simulink library "HEMERO"  (Simulink 3.00)
values from neighbouring files (symbols this model uses):
  K1 = 0.5    [ejh64.m]    (also in ejh65.m)
  K2 = 0.8    [ejh64.m]    (also in ejh65.m)
  x_camino = 0:0.01:10    [ejh64.m]    (also in ejh65.m)
  y_camino = x_camino.^2    [ejh64.m]    (also in ejh65.m)
undefined symbols (not defined in the file or in its folder): magnitude, nonlinear
libraries: simulink_extras x12, HEMERO x9, simulink3 x6, dspstat x4
(part 4 of 9)

== system HEMERO/Robots móviles/Control de robots móviles/Métodos basados en Teoría de Control/Seguimiento de caminos/Seguimiento de caminos (control lineal) ==
  v : Inport  Port=1  PortWidth=-1  SampleTime=-1  DataType=auto
      settings: SignalType=auto
  Configuracion síncrona : Subsystem
  Constant : Constant  Value=x_camino
  Constant1 : Constant  Value=y_camino
  Controlador lineal : Subsystem  Orientation=left
  Convertidor : Subsystem  Orientation=left
      mask Description: Este bloque permite transformar la salida del controlador a una señal que será adecuada al vehículo que se desea controlar
  Cálculo de parámetros : Subsystem
  x_vehículo : Outport  Port=1
  y_vehículo : Outport  Port=2
  phi_vehículo : Outport  Port=3
  wires:
  Constant/1 -> Cálculo de parámetros/1(x_camino)
  Constant1/1 -> Cálculo de parámetros/2(y_camino)
  Cálculo de parámetros/2(fi_gorro) -> Controlador lineal/1(fi_gorro), Convertidor/2(fi_gorro)
  Controlador lineal/1(u_cont) -> Convertidor/4(u_cont)
  Cálculo de parámetros/1(epsilon) -> Controlador lineal/3(epsilon)
  Convertidor/1(w) -> Configuracion síncrona/2(w)
  Configuracion síncrona/1(x_vehículo) -> Cálculo de parámetros/3(x_vehiculo), x_vehículo/1
  Configuracion síncrona/2(y_vehículo) -> Cálculo de parámetros/4(y_vehiculo), y_vehículo/1
  v/1 -> Configuracion síncrona/1(v), Controlador lineal/2(v), Convertidor/3(v)
  Cálculo de parámetros/3(R_c) -> Convertidor/1(R_c)
  Configuracion síncrona/3(phi_vehículo) -> Cálculo de parámetros/5(phi_vehiculo), phi_vehículo/1

== system HEMERO/Robots móviles/Control de robots móviles/Métodos basados en Teoría de Control/Seguimiento de caminos/Seguimiento de caminos (control no lineal) ==
  v : Inport  Port=1  PortWidth=-1  SampleTime=-1  DataType=auto
      settings: SignalType=auto
  " " : Subsystem  Orientation=left  mask{K2=K2}
      mask prompts: K2 "Parámetro K2:"
  Configuracion síncrona : Subsystem
  Constant : Constant  Value=x_camino
  Constant1 : Constant  Value=y_camino
  Controlador no lineal : Subsystem  Orientation=left
  Convertidor : Subsystem  Orientation=left
      mask Description: Este bloque permite transformar la salida del controlador a una señal que será adecuada al vehículo que se desea controlar
  Cálculo de parámetros : Subsystem
  x_vehículo : Outport  Port=1
  y_vehículo : Outport  Port=2
  phi_vehículo : Outport  Port=3
  wires:
  Constant/1 -> Cálculo de parámetros/1(x_camino)
  Constant1/1 -> Cálculo de parámetros/2(y_camino)
  Cálculo de parámetros/2(fi_gorro) -> Controlador no lineal/1(phi_gorro), Convertidor/2(fi_gorro)
  Controlador no lineal/1(u_cont) -> Convertidor/4(u_cont)
  Cálculo de parámetros/1(epsilon) -> Controlador no lineal/3(epsilon)
  Configuracion síncrona/1(x_vehículo) -> Cálculo de parámetros/3(x_vehiculo), x_vehículo/1
  Configuracion síncrona/2(y_vehículo) -> Cálculo de parámetros/4(y_vehiculo), y_vehículo/1
  v/1 -> Configuracion síncrona/1(v), Convertidor/3(v), Controlador no lineal/2(v), " "/1(v)
  Cálculo de parámetros/3(R_c) -> Convertidor/1(R_c)
  " "/1(k (v)) -> Controlador no lineal/4(k (v))
  Configuracion síncrona/3(phi_vehículo) -> Cálculo de parámetros/5(phi_vehiculo), phi_vehículo/1
  Convertidor/1(w) -> Configuracion síncrona/2(w)

== system HEMERO/Robots móviles/Control de robots móviles/Métodos basados en Teoría de Control/Seguimiento de trayectorias/Ejemplos ==
  Ejemplo H.6.6 : Subsystem
  Ejemplo H.6.7 : Subsystem
  Ejemplo H.6.8 : Subsystem

== system HEMERO/Robots móviles/Control de robots móviles/Métodos basados en Teoría de Control/Seguimiento de trayectorias/Seguimiento de trayectorias (Control lineal con escalado de velocidad) ==
  note: v
  note: w
  v_r : Inport  Port=1  PortWidth=-1  SampleTime=-1  DataType=auto
      settings: SignalType=auto
  w_r : Inport  Port=2  PortWidth=-1  SampleTime=-1  DataType=auto
      settings: SignalType=auto
  Cambio de variable : Subsystem
  Configuración síncrona referencia : Subsystem
  Configuración síncrona robot real : Subsystem
  Control lineal con escalado de velocidad : Subsystem
  Product : Product  Inputs=2  SaturateOnIntegerOverflow=on
  Sum : Sum  Inputs=-+  SaturateOnIntegerOverflow=on
  Sum1 : Sum  Inputs=+-  SaturateOnIntegerOverflow=on
  Trigonometric Function : Trigonometry  Operator=cos  OutputSignalType=auto
  v : Outport  Orientation=left  Port=1
  w : Outport  Orientation=left  Port=2
  x_ref : Outport  Port=3
  x : Outport  Port=4
  y_ref : Outport  Port=5
  y : Outport  Port=6
  phi_ref : Outport  Port=7
  phi : Outport  Port=8
  wires:
  v_r/1 -> Configuración síncrona referencia/1(v_r), Product/2, Control lineal con escalado de velocidad/4(v_r)
  Trigonometric Function/1 -> Product/1
  Product/1 -> Sum/2
  w_r/1 -> Configuración síncrona referencia/2(w_r), Sum1/1, Control lineal con escalado de velocidad/5(w_r)
  Sum1/1 -> Configuración síncrona robot real/2(w), w/1
  Sum/1 -> Configuración síncrona robot real/1(v), v/1
  Control lineal con escalado de velocidad/2(u2) -> Sum1/2
  Control lineal con escalado de velocidad/1(u1) -> Sum/1
  Cambio de variable/1(e1) -> Control lineal con escalado de velocidad/1(e1)
  Cambio de variable/2(e2) -> Control lineal con escalado de velocidad/2(e2)
  Cambio de variable/3(e3) -> Trigonometric Function/1, Control lineal con escalado de velocidad/3(e3)
  Configuración síncrona robot real/3(phi) -> Cambio de variable/6(phi), phi/1
  Configuración síncrona referencia/3(phi_r) -> Cambio de variable/5(phi_r), phi_ref/1
  Configuración síncrona robot real/2(y) -> Cambio de variable/4(y), y/1
  Configuración síncrona referencia/2(y_r) -> Cambio de variable/3(y_r), y_ref/1
  Configuración síncrona robot real/1(x) -> Cambio de variable/2(x), x/1
  Configuración síncrona referencia/1(x_r) -> Cambio de variable/1(x_r), x_ref/1

== system HEMERO/Robots móviles/Control de robots móviles/Métodos basados en Teoría de Control/Seguimiento de trayectorias/Seguimiento de trayectorias (Control lineal) ==
  note: v
  note: w
  v_r : Inport  Port=1  PortWidth=-1  SampleTime=-1  DataType=auto
      settings: SignalType=auto
  w_r : Inport  Port=2  PortWidth=-1  SampleTime=-1  DataType=auto
      settings: SignalType=auto
  Cambio de variable : Subsystem
  Configuración síncrona referencia : Subsystem
  Configuración síncrona robot real : Subsystem
  Control lineal : Subsystem
  Product : Product  Inputs=2  SaturateOnIntegerOverflow=on
  Sum : Sum  Inputs=-+  SaturateOnIntegerOverflow=on
  Sum1 : Sum  Inputs=+-  SaturateOnIntegerOverflow=on
  Trigonometric Function : Trigonometry  Operator=cos  OutputSignalType=auto
  v : Outport  Orientation=left  Port=1
  w : Outport  Orientation=left  Port=2
  x_ref : Outport  Port=3
  x : Outport  Port=4
  y_ref : Outport  Port=5
  y : Outport  Port=6
  phi_ref : Outport  Port=7
  phi : Outport  Port=8
  wires:
  v_r/1 -> Configuración síncrona referencia/1(v_r), Product/2, Control lineal/4(v_r)
  Trigonometric Function/1 -> Product/1
  Product/1 -> Sum/2
  w_r/1 -> Configuración síncrona referencia/2(w_r), Sum1/1
  Sum1/1 -> Configuración síncrona robot real/2(w), w/1
  Sum/1 -> Configuración síncrona robot real/1(v), v/1
  Control lineal/2(u2) -> Sum1/2
  Control lineal/1(u1) -> Sum/1
  Cambio de variable/1(e1) -> Control lineal/1(e1)
  Cambio de variable/2(e2) -> Control lineal/2(e2)
  Cambio de variable/3(e3) -> Trigonometric Function/1, Control lineal/3(e3)
  Configuración síncrona referencia/1(x_r) -> Cambio de variable/1(x_r), x_ref/1
  Configuración síncrona robot real/1(x) -> Cambio de variable/2(x), x/1
  Configuración síncrona referencia/2(y_r) -> Cambio de variable/3(y_r), y_ref/1
  Configuración síncrona robot real/2(y) -> Cambio de variable/4(y), y/1
  Configuración síncrona referencia/3(phi_r) -> Cambio de variable/5(phi_r), phi_ref/1
  Configuración síncrona robot real/3(phi) -> Cambio de variable/6(phi), phi/1

== system HEMERO/Robots móviles/Control de robots móviles/Métodos basados en Teoría de Control/Seguimiento de trayectorias/Seguimiento de trayectorias (Control no lineal) ==
  note: v
  note: w
  v_r : Inport  Port=1  PortWidth=-1  SampleTime=-1  DataType=auto
      settings: SignalType=auto
  w_r : Inport  Port=2  PortWidth=-1  SampleTime=-1  DataType=auto
      settings: SignalType=auto
  " " : Trigonometry  Operator=cos  OutputSignalType=auto
  Cambio de variable : Subsystem
  Configuración síncrona referencia : Subsystem
  Configuración síncrona robot real : Subsystem
  Control no lineal : Subsystem
  Cálculo de K1 y K3 : Subsystem
  Product : Product  Inputs=2  SaturateOnIntegerOverflow=on
  Sum : Sum  Inputs=-+  SaturateOnIntegerOverflow=on
  Sum1 : Sum  Inputs=+-  SaturateOnIntegerOverflow=on
  v : Outport  Orientation=left  Port=1
  w : Outport  Orientation=left  Port=2
  x_ref : Outport  Port=3
  x : Outport  Port=4
  y_ref : Outport  Port=5
  y : Outport  Port=6
  phi_ref : Outport  Port=7
  phi : Outport  Port=8
  wires:
  v_r/1 -> Configuración síncrona referencia/1(v_r), Product/2, Control no lineal/4(v_r), Cálculo de K1 y K3/2(v_r)
  " "/1 -> Product/1
  Product/1 -> Sum/2
  w_r/1 -> Configuración síncrona referencia/2(w_r), Sum1/1, Cálculo de K1 y K3/1(w_r)
  Sum1/1 -> Configuración síncrona robot real/2(w), w/1
  Sum/1 -> Configuración síncrona robot real/1(v), v/1
  Control no lineal/2(u2) -> Sum1/2
  Control no lineal/1(u1) -> Sum/1
  Cambio de variable/1(e1) -> Control no lineal/1(e1)
  Cambio de variable/2(e2) -> Control no lineal/2(e2)
  Cambio de variable/3(e3) -> " "/1, Control no lineal/3(e3)
  Cálculo de K1 y K3/1(K1) -> Control no lineal/5(K1), Control no lineal/6(K3)
  Configuración síncrona robot real/3(phi) -> Cambio de variable/6(phi), phi/1
  Configuración síncrona referencia/1(x_r) -> Cambio de variable/1(x_r), x_ref/1
  Configuración síncrona robot real/1(x) -> Cambio de variable/2(x), x/1
  Configuración síncrona referencia/2(y_r) -> Cambio de variable/3(y_r), y_ref/1
  Configuración síncrona robot real/2(y) -> Cambio de variable/4(y), y/1
  Configuración síncrona referencia/3(phi_r) -> Cambio de variable/5(phi_r), phi_ref/1

== system HEMERO/Robots manipuladores base fija/Control basado en el modelo/Control Adaptativo/Ejemplos/Ejemplo H.5.5/Control PD ==
  qd : Inport  Port=1  PortWidth=-1  SampleTime=-1  DataType=auto
      settings: SignalType=auto
  q : Inport  Port=2  PortWidth=-1  SampleTime=-1  DataType=auto
      settings: SignalType=auto
  qd' : Inport  Port=3  PortWidth=-1  SampleTime=-1  DataType=auto
      settings: SignalType=auto
  q' : Inport  Port=4  PortWidth=-1  SampleTime=-1  DataType=auto
      settings: SignalType=auto
  A : StateSpace  A=[]  B=[]  C=[]  D=K  X0=0  mask(Matrix Gain){@1=A}
      mask prompts: @1 "Gain matrix:"
      mask help: Matrix Gain.
      mask init:
      | K=@1;
      mask Help: Multiplies input vector by entered matrix to produce output vector (y=Au).
      mask Display: disp('K')
  Kv : StateSpace  A=[]  B=[]  C=[]  D=K  X0=0  mask(Matrix Gain){@1=Kv}
      mask prompts: @1 "Gain matrix:"
      mask help: Matrix Gain.
      mask init:
      | K=@1;
      mask Help: Multiplies input vector by entered matrix to produce output vector (y=Au).
      mask Display: disp('K')
  Kv1 : StateSpace  A=[]  B=[]  C=[]  D=K  X0=0  mask(Matrix Gain){@1=Kv}
      mask prompts: @1 "Gain matrix:"
      mask help: Matrix Gain.
      mask init:
      | K=@1;
      mask Help: Multiplies input vector by entered matrix to produce output vector (y=Au).
      mask Display: disp('K')
  Sum : Sum  Inputs=+-  SaturateOnIntegerOverflow=on
  Sum1 : Sum  Inputs=+-  SaturateOnIntegerOverflow=on
  Sum2 : Sum  Inputs=++  SaturateOnIntegerOverflow=on
  tau_r : Outport  Port=1  InitialOutput=0
  wires:
  Sum2/1 -> tau_r/1
  Kv1/1 -> Sum2/1
  Kv/1 -> Sum2/2
  Sum1/1 -> Kv/1
  q'/1 -> Sum1/2
  qd'/1 -> Sum1/1
  q/1 -> Sum/2
  qd/1 -> Sum/1
  Sum/1 -> A/1
  A/1 -> Kv1/1

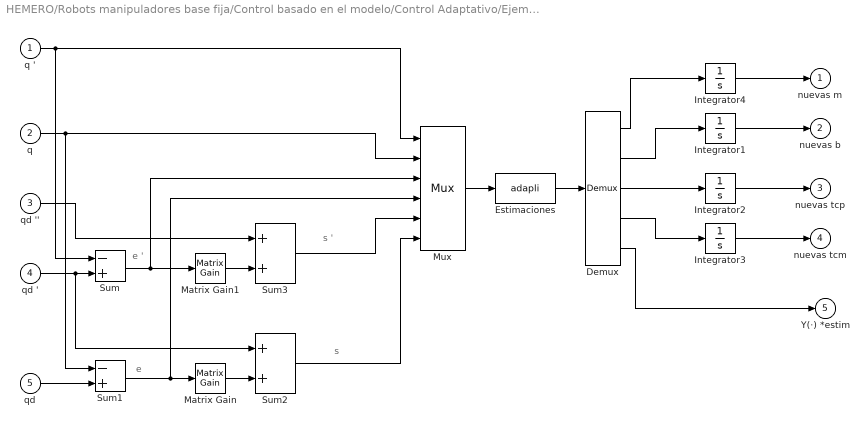
== system HEMERO/Robots manipuladores base fija/Control basado en el modelo/Control Adaptativo/Ejemplos/Ejemplo H.5.5/Control de inercia adaptativo ==
  note: e
  note: e '
  note: s
  note: s '
  q ' : Inport  Port=1  PortWidth=-1  SampleTime=-1  DataType=auto
      settings: SignalType=auto
  q : Inport  Port=2  PortWidth=-1  SampleTime=-1  DataType=auto
      settings: SignalType=auto
  qd '' : Inport  Port=3  PortWidth=-1  SampleTime=-1  DataType=auto
      settings: SignalType=auto
  qd ' : Inport  Port=4  PortWidth=-1  SampleTime=-1  DataType=auto
      settings: SignalType=auto
  qd : Inport  Port=5  PortWidth=-1  SampleTime=-1  DataType=auto
      settings: SignalType=auto
  Demux : Demux  Outputs=5
  Estimaciones : S-Function  FunctionName=adapli  Parameters=dyn, gamma, a, grav  PortCounts=[]  SFunctionModules=''
  Integrator1 : Integrator  ExternalReset=none  InitialConditionSource=internal  InitialCondition=b_inicial(:)  LimitOutput=off  UpperSaturationLimit=inf  LowerSaturationLimit=-inf  ShowSaturationPort=off  ShowStatePort=off  AbsoluteTolerance=auto
  Integrator2 : Integrator  ExternalReset=none  InitialConditionSource=internal  InitialCondition=tcp_inicial(:)  LimitOutput=off  UpperSaturationLimit=inf  LowerSaturationLimit=-inf  ShowSaturationPort=off  ShowStatePort=off  AbsoluteTolerance=auto
  Integrator3 : Integrator  ExternalReset=none  InitialConditionSource=internal  InitialCondition=tcm_inicial(:)  LimitOutput=off  UpperSaturationLimit=inf  LowerSaturationLimit=-inf  ShowSaturationPort=off  ShowStatePort=off  AbsoluteTolerance=auto
  Integrator4 : Integrator  ExternalReset=none  InitialConditionSource=internal  InitialCondition=m_inicial(:)  LimitOutput=off  UpperSaturationLimit=inf  LowerSaturationLimit=-inf  ShowSaturationPort=off  ShowStatePort=off  AbsoluteTolerance=auto
  Matrix Gain : simulink3/Math/Matrix Gain  K=a
  Matrix Gain1 : simulink3/Math/Matrix Gain  K=a
  Mux : Mux  Inputs=6
      settings: DisplayOption=none
  Sum : Sum  Inputs=-+  SaturateOnIntegerOverflow=on
  Sum1 : Sum  Inputs=-+  SaturateOnIntegerOverflow=on
  Sum2 : Sum  Inputs=++  SaturateOnIntegerOverflow=on
  Sum3 : Sum  Inputs=++  SaturateOnIntegerOverflow=on
  nuevas m : Outport  Port=1  InitialOutput=0
  nuevas b : Outport  Port=2  InitialOutput=0
  nuevas tcp : Outport  Port=3  InitialOutput=0
  nuevas tcm : Outport  Port=4  InitialOutput=0
  Y(·) *estim : Outport  Port=5  InitialOutput=0
  wires:
  q '/1 -> Mux/1, Sum/1
  q/1 -> Mux/2, Sum1/1
  Mux/1 -> Estimaciones/1
  Estimaciones/1 -> Demux/1
  Demux/2 -> Integrator1/1
  Integrator1/1 -> nuevas b/1
  Demux/3 -> Integrator2/1
  Integrator2/1 -> nuevas tcp/1
  Demux/4 -> Integrator3/1
  Integrator3/1 -> nuevas tcm/1
  qd/1 -> Sum1/2
  Matrix Gain/1 -> Sum2/2
  qd '/1 -> Sum/2, Sum2/1
  Matrix Gain1/1 -> Sum3/2
  qd ''/1 -> Sum3/1
  Sum2/1 -> Mux/6
  Sum3/1 -> Mux/5
  Sum/1 -> Matrix Gain1/1, Mux/3
  Sum1/1 -> Matrix Gain/1, Mux/4
  Demux/5 -> Y(·) *estim/1
  Demux/1 -> Integrator4/1
  Integrator4/1 -> nuevas m/1

== system HEMERO/Robots manipuladores base fija/Control basado en el modelo/Control Adaptativo/Ejemplos/Ejemplo H.5.5/Inversa de la matriz de masas real ==
  q : Inport  Port=1  PortWidth=-1  SampleTime=-1  DataType=auto
      settings: SignalType=auto
  In : Inport  Port=2  PortWidth=-1  SampleTime=-1  DataType=auto
      settings: SignalType=auto
  Masas : S-Function  FunctionName=sminv  Parameters=dyn  PortCounts=[]  SFunctionModules=''
  Mux : Mux  Inputs=2
      settings: DisplayOption=none
  M(q)^(-1) · In : Outport  Port=1  InitialOutput=0
  wires:
  Mux/1 -> Masas/1
  q/1 -> Mux/1
  In/1 -> Mux/2
  Masas/1 -> M(q)^(-1) · In/1

== system HEMERO/Robots manipuladores base fija/Control basado en el modelo/Control Adaptativo/Ejemplos/Ejemplo H.5.5/Término gravitatorio estimado ==
  q : Inport  Port=1  PortWidth=-1  SampleTime=-1  DataType=auto
      settings: SignalType=auto
  nuevas m : Inport  Port=2  PortWidth=-1  SampleTime=-1  DataType=auto
      settings: SignalType=auto
  Gravedad : S-Function  FunctionName=esgravity  Parameters=dyn,grav  PortCounts=[]  SFunctionModules=''
  Mux : Mux  Inputs=2
      settings: DisplayOption=none
  G (q) : Outport  Port=1  InitialOutput=0
  wires:
  Mux/1 -> Gravedad/1
  nuevas m/1 -> Mux/2
  q/1 -> Mux/1
  Gravedad/1 -> G (q)/1

== system HEMERO/Robots manipuladores base fija/Control basado en el modelo/Control Adaptativo/Ejemplos/Ejemplo H.5.5/Término gravitatorio real ==
  q : Inport  Port=1  PortWidth=-1  SampleTime=-1  DataType=auto
      settings: SignalType=auto
  Gravedad : S-Function  FunctionName=sgravity  Parameters=dyn,grav  PortCounts=[]  SFunctionModules=''
  G (q) : Outport  Port=1  InitialOutput=0
  wires:
  q/1 -> Gravedad/1
  Gravedad/1 -> G (q)/1

== system HEMERO/Robots manipuladores base fija/Control basado en el modelo/Control Adaptativo/Ejemplos/Ejemplo H.5.5/Término Vm de Coriolis estimado ==
  q : Inport  Port=1  PortWidth=-1  SampleTime=-1  DataType=auto
      settings: SignalType=auto
  q ' : Inport  Port=2  PortWidth=-1  SampleTime=-1  DataType=auto
      settings: SignalType=auto
  In : Inport  Port=3  PortWidth=-1  SampleTime=-1  DataType=auto
      settings: SignalType=auto
  nuevas m : Inport  Port=4  PortWidth=-1  SampleTime=-1  DataType=auto
      settings: SignalType=auto
  "  " : S-Function  FunctionName=esvmcorioli  Parameters=dyn  PortCounts=[]  SFunctionModules=''
  Mux : Mux  Inputs=4
      settings: DisplayOption=none
  Vm (q,q')·In : Outport  Port=1  InitialOutput=0
  wires:
  nuevas m/1 -> Mux/4
  "  "/1 -> Vm (q,q')·In/1
  Mux/1 -> "  "/1
  In/1 -> Mux/3
  q/1 -> Mux/1
  q '/1 -> Mux/2

== system HEMERO/Robots manipuladores base fija/Control basado en el modelo/Control Adaptativo/Ejemplos/Ejemplo H.5.5/Término de la matriz de masas estimado ==
  q : Inport  Port=1  PortWidth=-1  SampleTime=-1  DataType=auto
      settings: SignalType=auto
  In : Inport  Port=2  PortWidth=-1  SampleTime=-1  DataType=auto
      settings: SignalType=auto
  nuevas m : Inport  Port=3  PortWidth=-1  SampleTime=-1  DataType=auto
      settings: SignalType=auto
  Masas : S-Function  FunctionName=esinertia  Parameters=dyn  PortCounts=[]  SFunctionModules=''
  Mux : Mux  Inputs=3
      settings: DisplayOption=none
  M (q)·In : Outport  Port=1  InitialOutput=0
  wires:
  nuevas m/1 -> Mux/3
  Masas/1 -> M (q)·In/1
  Mux/1 -> Masas/1
  q/1 -> Mux/1
  In/1 -> Mux/2

== system HEMERO/Robots manipuladores base fija/Control basado en el modelo/Control Adaptativo/Ejemplos/Ejemplo H.5.5/Términos centrífugos y de Coriolis reales ==
  q : Inport  Port=1  PortWidth=-1  SampleTime=-1  DataType=auto
      settings: SignalType=auto
  q' : Inport  Port=2  PortWidth=-1  SampleTime=-1  DataType=auto
      settings: SignalType=auto
  Centrífugos y Coriolis : S-Function  FunctionName=scoriolis  Parameters=dyn  PortCounts=[]  SFunctionModules=''
  Mux : Mux  Inputs=2
      settings: DisplayOption=none
  V (q,q') : Outport  Port=1  InitialOutput=0
  wires:
  Mux/1 -> Centrífugos y Coriolis/1
  q/1 -> Mux/1
  q'/1 -> Mux/2
  Centrífugos y Coriolis/1 -> V (q,q')/1

== system HEMERO/Robots manipuladores base fija/Control basado en el modelo/Control con aprendizaje/Ejemplos/Ejemplo H.5.1/Control PD ==
  qd : Inport  Port=1  PortWidth=-1  SampleTime=-1  DataType=auto
      settings: SignalType=auto
  q : Inport  Port=2  PortWidth=-1  SampleTime=-1  DataType=auto
      settings: SignalType=auto
  qd' : Inport  Port=3  PortWidth=-1  SampleTime=-1  DataType=auto
      settings: SignalType=auto
  q' : Inport  Port=4  PortWidth=-1  SampleTime=-1  DataType=auto
      settings: SignalType=auto
  qd'' : Inport  Port=5  PortWidth=-1  SampleTime=-1  DataType=auto
      settings: SignalType=auto
  Kp : StateSpace  A=[]  B=[]  C=[]  D=K  X0=0  mask(Matrix Gain){@1=Kp}
      mask prompts: @1 "Gain matrix:"
      mask help: Matrix Gain.
      mask init:
      | K=@1;
      mask Help: Multiplies input vector by entered matrix to produce output vector (y=Au).
      mask Display: disp('K')
  Kv : StateSpace  A=[]  B=[]  C=[]  D=K  X0=0  mask(Matrix Gain){@1=Kv}
      mask prompts: @1 "Gain matrix:"
      mask help: Matrix Gain.
      mask init:
      | K=@1;
      mask Help: Multiplies input vector by entered matrix to produce output vector (y=Au).
      mask Display: disp('K')
  Sum : Sum  Inputs=+-  SaturateOnIntegerOverflow=on
  Sum1 : Sum  Inputs=+-  SaturateOnIntegerOverflow=on
  Sum2 : Sum  Inputs=+++  SaturateOnIntegerOverflow=on
  tau_r : Outport  Port=1  InitialOutput=0
  wires:
  Sum2/1 -> tau_r/1
  qd''/1 -> Sum2/3
  Kp/1 -> Sum2/1
  Kv/1 -> Sum2/2
  Sum1/1 -> Kv/1
  Sum/1 -> Kp/1
  q'/1 -> Sum1/2
  qd'/1 -> Sum1/1
  q/1 -> Sum/2
  qd/1 -> Sum/1

== system HEMERO/Robots manipuladores base fija/Control basado en el modelo/Control con aprendizaje/Ejemplos/Ejemplo H.5.1/Modelo del robot ==
  note: q
  note: q''
  note: q'
  tau : Inport  Port=1  PortWidth=-1  SampleTime=-1  DataType=auto
      settings: SignalType=auto
  Integrator : Integrator  ExternalReset=none  InitialConditionSource=internal  InitialCondition=inivel(:)  LimitOutput=off  UpperSaturationLimit=inf  LowerSaturationLimit=-inf  ShowSaturationPort=off  ShowStatePort=off  AbsoluteTolerance=auto
  Integrator1 : Integrator  ExternalReset=none  InitialConditionSource=internal  InitialCondition=inipos(:)  LimitOutput=off  UpperSaturationLimit=inf  LowerSaturationLimit=-inf  ShowSaturationPort=off  ShowStatePort=off  AbsoluteTolerance=auto
  Inversa de la matriz de masas : HEMERO/Robots manipuladores base fija/Modelo Dinámico/Trayectorias articulares/Inversa de la matriz de masas  dyn=dyn
  Modelo de fricciones : HEMERO/Robots manipuladores base fija/Modelo Dinámico/Trayectorias articulares/Modelo de fricciones  G=dyn (:,17)  b=dyn (:,18)  tcp=dyn (:,19)  tcm=dyn (:,20)
  Sum : Sum  Inputs=+---  SaturateOnIntegerOverflow=on
  Términos gravitatorios : HEMERO/Robots manipuladores base fija/Modelo Dinámico/Trayectorias articulares/Términos gravitatorios  dyn=dyn  grav=grav
  Términos centrífugos y de Coriolis : HEMERO/Robots manipuladores base fija/Modelo Dinámico/Trayectorias articulares/Términos centrífugos y de Coriolis  dyn=dyn
  q : Outport  Port=1  InitialOutput=0
  q' : Outport  Port=2  InitialOutput=0
  q'' : Outport  Port=3  InitialOutput=0
  wires:
  Integrator1/1 -> q/1, Inversa de la matriz de masas/1, Términos centrífugos y de Coriolis/1, Términos gravitatorios/1
  Integrator/1 -> Integrator1/1, q'/1, Términos centrífugos y de Coriolis/2, Modelo de fricciones/1
  Sum/1 -> Inversa de la matriz de masas/2
  tau/1 -> Sum/1
  Inversa de la matriz de masas/1 -> Integrator/1, q''/1
  Términos gravitatorios/1 -> Sum/4
  Términos centrífugos y de Coriolis/1 -> Sum/3
  Modelo de fricciones/1 -> Sum/2

== system HEMERO/Robots manipuladores base fija/Control basado en el modelo/Control con aprendizaje/Ejemplos/Ejemplo H.5.1/Par realimentado aprendido ==
  note: e ''
  note: e '
  note: e
  qd '' : Inport  Port=1  PortWidth=-1  SampleTime=-1  DataType=auto
      settings: SignalType=auto
  q '' : Inport  Port=2  PortWidth=-1  SampleTime=-1  DataType=auto
      settings: SignalType=auto
  qd ' : Inport  Port=3  PortWidth=-1  SampleTime=-1  DataType=auto
      settings: SignalType=auto
  q ' : Inport  Port=4  PortWidth=-1  SampleTime=-1  DataType=auto
      settings: SignalType=auto
  qd : Inport  Port=5  PortWidth=-1  SampleTime=-1  DataType=auto
      settings: SignalType=auto
  q : Inport  Port=6  PortWidth=-1  SampleTime=-1  DataType=auto
      settings: SignalType=auto
  Demux : Demux  Outputs=4
  Mux : Mux  Inputs=3
      settings: DisplayOption=none
  S-Function : S-Function  FunctionName=learn  Parameters=Kp, Kv, mu, tfinal  PortCounts=[]  SFunctionModules=''
  Sum : Sum  Inputs=+-  SaturateOnIntegerOverflow=on
  Sum1 : Sum  Inputs=+-  SaturateOnIntegerOverflow=on
  Sum2 : Sum  Inputs=+-  SaturateOnIntegerOverflow=on
  To Workspace1 : ToWorkspace  VariableName=error  SampleTime=-1  SaveFormat=Matrix
  To Workspace2 : ToWorkspace  VariableName=error_d  SampleTime=-1  SaveFormat=Matrix
  To Workspace3 : ToWorkspace  VariableName=error_dd  SampleTime=-1  SaveFormat=Matrix
  To Workspace4 : ToWorkspace  VariableName=edd  SampleTime=-1  SaveFormat=Matrix
  To Workspace5 : ToWorkspace  VariableName=dknueva  SampleTime=-1  SaveFormat=Matrix
  To Workspace6 : ToWorkspace  VariableName=ed  SampleTime=-1  SaveFormat=Matrix
  To Workspace7 : ToWorkspace  VariableName=e  SampleTime=-1  SaveFormat=Matrix
  Término de la matriz de masas estimado : Subsystem  mask(Término asociado a la matriz de masas){dyn=dyn}
      mask prompts: dyn "Matriz de parámetros cinemáticos y dinámicos:"
      mask help: Este bloque calcula el par correspondiente al término en el que aparece la matriz de masas.
  gamma (k) : Outport  Port=1
  wires:
  Mux/1 -> S-Function/1
  S-Function/1 -> Demux/1
  qd ''/1 -> Sum/1
  q ''/1 -> Sum/2
  qd '/1 -> Sum1/1
  q '/1 -> Sum1/2
  qd/1 -> Sum2/1
  Demux/1 -> Término de la matriz de masas estimado/2(In), To Workspace5/1
  Sum2/1 -> Mux/3, To Workspace7/1
  Sum1/1 -> Mux/2, To Workspace6/1
  Sum/1 -> Mux/1, To Workspace4/1
  Demux/2 -> To Workspace1/1
  Demux/3 -> To Workspace2/1
  Demux/4 -> To Workspace3/1
  q/1 -> Sum2/2, Término de la matriz de masas estimado/1(q)
  Término de la matriz de masas estimado/1(M (q)·In) -> gamma (k)/1

== system HEMERO/Robots manipuladores base fija/Control basado en el modelo/Control con aprendizaje/Ejemplos/Ejemplo H.5.1/Término de la matriz de masas ==
  q : Inport  Port=1  PortWidth=-1  SampleTime=-1  DataType=auto
      settings: SignalType=auto
  In : Inport  Port=2  PortWidth=-1  SampleTime=-1  DataType=auto
      settings: SignalType=auto
  Masas : S-Function  FunctionName=sinertia  Parameters=dyn  PortCounts=[]  SFunctionModules=''
  Mux : Mux  Inputs=2
      settings: DisplayOption=none
  M (q)·In : Outport  Port=1  InitialOutput=0
  wires:
  Masas/1 -> M (q)·In/1
  In/1 -> Mux/2
  q/1 -> Mux/1
  Mux/1 -> Masas/1

== system HEMERO/Robots manipuladores base fija/Control basado en el modelo/Control con aprendizaje/Ejemplos/Ejemplo H.5.1/Términos gravitatorios ==
  q : Inport  Port=1  PortWidth=-1  SampleTime=-1  DataType=auto
      settings: SignalType=auto
  Gravedad : S-Function  FunctionName=sgravity  Parameters=dyn,grav  PortCounts=[]  SFunctionModules=''
  G (q) : Outport  Port=1  InitialOutput=0
  wires:
  Gravedad/1 -> G (q)/1
  q/1 -> Gravedad/1

== system HEMERO/Robots manipuladores base fija/Control basado en el modelo/Control con aprendizaje/Ejemplos/Ejemplo H.5.1/Términos centrífugos y de Coriolis ==
  q : Inport  Port=1  PortWidth=-1  SampleTime=-1  DataType=auto
      settings: SignalType=auto
  q' : Inport  Port=2  PortWidth=-1  SampleTime=-1  DataType=auto
      settings: SignalType=auto
  Centrífugos y Coriolis : S-Function  FunctionName=scoriolis  Parameters=dyn  PortCounts=[]  SFunctionModules=''
  Mux : Mux  Inputs=2
      settings: DisplayOption=none
  V (q,q') : Outport  Port=1  InitialOutput=0
  wires:
  Centrífugos y Coriolis/1 -> V (q,q')/1
  q'/1 -> Mux/2
  q/1 -> Mux/1
  Mux/1 -> Centrífugos y Coriolis/1

== system HEMERO/Robots manipuladores base fija/Control basado en el modelo/Par Computado/Ejemplos/Ejemplo H.5.2/Control PD ==
  qd : Inport  Port=1  PortWidth=-1  SampleTime=-1  DataType=auto
      settings: SignalType=auto
  q : Inport  Port=2  PortWidth=-1  SampleTime=-1  DataType=auto
      settings: SignalType=auto
  qd' : Inport  Port=3  PortWidth=-1  SampleTime=-1  DataType=auto
      settings: SignalType=auto
  q' : Inport  Port=4  PortWidth=-1  SampleTime=-1  DataType=auto
      settings: SignalType=auto
  qd'' : Inport  Port=5  PortWidth=-1  SampleTime=-1  DataType=auto
      settings: SignalType=auto
  Kp : StateSpace  A=[]  B=[]  C=[]  D=K  X0=0  mask(Matrix Gain){@1=Kp}
      mask prompts: @1 "Gain matrix:"
      mask help: Matrix Gain.
      mask init:
      | K=@1;
      mask Help: Multiplies input vector by entered matrix to produce output vector (y=Au).
      mask Display: disp('K')
  Kv : StateSpace  A=[]  B=[]  C=[]  D=K  X0=0  mask(Matrix Gain){@1=Kv}
      mask prompts: @1 "Gain matrix:"
      mask help: Matrix Gain.
      mask init:
      | K=@1;
      mask Help: Multiplies input vector by entered matrix to produce output vector (y=Au).
      mask Display: disp('K')
  Sum : Sum  Inputs=+-  SaturateOnIntegerOverflow=on
  Sum1 : Sum  Inputs=+-  SaturateOnIntegerOverflow=on
  Sum2 : Sum  Inputs=+++  SaturateOnIntegerOverflow=on
  tau_r : Outport  Port=1  InitialOutput=0
  wires:
  qd/1 -> Sum/1
  q/1 -> Sum/2
  qd'/1 -> Sum1/1
  q'/1 -> Sum1/2
  Sum/1 -> Kp/1
  Sum1/1 -> Kv/1
  Kv/1 -> Sum2/2
  Kp/1 -> Sum2/1
  qd''/1 -> Sum2/3
  Sum2/1 -> tau_r/1

== system HEMERO/Robots manipuladores base fija/Control basado en el modelo/Par Computado/Ejemplos/Ejemplo H.5.2/Estimada1 ==
  q : Inport  Port=1  PortWidth=-1  SampleTime=-1  DataType=auto
      settings: SignalType=auto
  Gravedad : S-Function  FunctionName=sgravity  Parameters=dyn,grav  PortCounts=[]  SFunctionModules=''
  G (q) : Outport  Port=1  InitialOutput=0
  wires:
  q/1 -> Gravedad/1
  Gravedad/1 -> G (q)/1

== system HEMERO/Robots manipuladores base fija/Control basado en el modelo/Par Computado/Ejemplos/Ejemplo H.5.2/Estimada2 ==
  q : Inport  Port=1  PortWidth=-1  SampleTime=-1  DataType=auto
      settings: SignalType=auto
  In : Inport  Port=2  PortWidth=-1  SampleTime=-1  DataType=auto
      settings: SignalType=auto
  Masas : S-Function  FunctionName=sinertia  Parameters=dyn  PortCounts=[]  SFunctionModules=''
  Mux : Mux  Inputs=2
      settings: DisplayOption=none
  M (q)·In : Outport  Port=1  InitialOutput=0
  wires:
  Mux/1 -> Masas/1
  q/1 -> Mux/1
  In/1 -> Mux/2
  Masas/1 -> M (q)·In/1

== system HEMERO/Robots manipuladores base fija/Control basado en el modelo/Par Computado/Ejemplos/Ejemplo H.5.2/Estimada3 ==
  q : Inport  Port=1  PortWidth=-1  SampleTime=-1  DataType=auto
      settings: SignalType=auto
  q' : Inport  Port=2  PortWidth=-1  SampleTime=-1  DataType=auto
      settings: SignalType=auto
  Centrífugos y Coriolis : S-Function  FunctionName=scoriolis  Parameters=dyn  PortCounts=[]  SFunctionModules=''
  Mux : Mux  Inputs=2
      settings: DisplayOption=none
  V (q,q') : Outport  Port=1  InitialOutput=0
  wires:
  Mux/1 -> Centrífugos y Coriolis/1
  q/1 -> Mux/1
  q'/1 -> Mux/2
  Centrífugos y Coriolis/1 -> V (q,q')/1

== system HEMERO/Robots manipuladores base fija/Control basado en el modelo/Par Computado/Ejemplos/Ejemplo H.5.2/Real1 ==
  q : Inport  Port=1  PortWidth=-1  SampleTime=-1  DataType=auto
      settings: SignalType=auto
  q' : Inport  Port=2  PortWidth=-1  SampleTime=-1  DataType=auto
      settings: SignalType=auto
  Centrífugos y Coriolis : S-Function  FunctionName=scoriolis  Parameters=dyn  PortCounts=[]  SFunctionModules=''
  Mux : Mux  Inputs=2
      settings: DisplayOption=none
  V (q,q') : Outport  Port=1  InitialOutput=0
  wires:
  Mux/1 -> Centrífugos y Coriolis/1
  q/1 -> Mux/1
  q'/1 -> Mux/2
  Centrífugos y Coriolis/1 -> V (q,q')/1

== system HEMERO/Robots manipuladores base fija/Control basado en el modelo/Par Computado/Ejemplos/Ejemplo H.5.2/Real2 ==
  q : Inport  Port=1  PortWidth=-1  SampleTime=-1  DataType=auto
      settings: SignalType=auto
  Gravedad : S-Function  FunctionName=sgravity  Parameters=dyn,grav  PortCounts=[]  SFunctionModules=''
  G (q) : Outport  Port=1  InitialOutput=0
  wires:
  q/1 -> Gravedad/1
  Gravedad/1 -> G (q)/1

== system HEMERO/Robots manipuladores base fija/Control basado en el modelo/Par Computado/Ejemplos/Ejemplo H.5.2/Real3 ==
  q : Inport  Port=1  PortWidth=-1  SampleTime=-1  DataType=auto
      settings: SignalType=auto
  In : Inport  Port=2  PortWidth=-1  SampleTime=-1  DataType=auto
      settings: SignalType=auto
  Masas : S-Function  FunctionName=sminv  Parameters=dyn  PortCounts=[]  SFunctionModules=''
  Mux : Mux  Inputs=2
      settings: DisplayOption=none
  M(q)^(-1) · In : Outport  Port=1  InitialOutput=0
  wires:
  Mux/1 -> Masas/1
  q/1 -> Mux/1
  In/1 -> Mux/2
  Masas/1 -> M(q)^(-1) · In/1

== system HEMERO/Robots manipuladores base fija/Control basado en el modelo/Par Computado/Ejemplos/Ejemplo H.5.3/Control PD ==
  qd : Inport  Port=1  PortWidth=-1  SampleTime=-1  DataType=auto
      settings: SignalType=auto
  q : Inport  Port=2  PortWidth=-1  SampleTime=-1  DataType=auto
      settings: SignalType=auto
  qd' : Inport  Port=3  PortWidth=-1  SampleTime=-1  DataType=auto
      settings: SignalType=auto
  q' : Inport  Port=4  PortWidth=-1  SampleTime=-1  DataType=auto
      settings: SignalType=auto
  qd'' : Inport  Port=5  PortWidth=-1  SampleTime=-1  DataType=auto
      settings: SignalType=auto
  Kp : HEMERO/Robots manipuladores base fija/Control basado en el modelo/Par Computado/Ejemplos/Ejemplo H.5.2/Control PD/Kp  MaskParam1=Kp
  Kv : HEMERO/Robots manipuladores base fija/Control basado en el modelo/Par Computado/Ejemplos/Ejemplo H.5.2/Control PD/Kv  MaskParam1=Kv
  Sum : Sum  Inputs=+-  SaturateOnIntegerOverflow=on
  Sum1 : Sum  Inputs=+-  SaturateOnIntegerOverflow=on
  Sum2 : Sum  Inputs=+++  SaturateOnIntegerOverflow=on
  tau_r : Outport  Port=1  InitialOutput=0
  wires:
  qd/1 -> Sum/1
  q/1 -> Sum/2
  qd'/1 -> Sum1/1
  q'/1 -> Sum1/2
  Sum/1 -> Kp/1
  Sum1/1 -> Kv/1
  Kv/1 -> Sum2/2
  Kp/1 -> Sum2/1
  qd''/1 -> Sum2/3
  Sum2/1 -> tau_r/1

== system HEMERO/Robots manipuladores base fija/Control basado en el modelo/Par Computado/Ejemplos/Ejemplo H.5.3/Estimada1 ==
  q : Inport  Port=1  PortWidth=-1  SampleTime=-1  DataType=auto
      settings: SignalType=auto
  Gravedad : S-Function  FunctionName=sgravity  Parameters=dyn,grav  PortCounts=[]  SFunctionModules=''
  G (q) : Outport  Port=1  InitialOutput=0
  wires:
  q/1 -> Gravedad/1
  Gravedad/1 -> G (q)/1

== system HEMERO/Robots manipuladores base fija/Control basado en el modelo/Par Computado/Ejemplos/Ejemplo H.5.3/Estimada2 ==
  q : Inport  Port=1  PortWidth=-1  SampleTime=-1  DataType=auto
      settings: SignalType=auto
  In : Inport  Port=2  PortWidth=-1  SampleTime=-1  DataType=auto
      settings: SignalType=auto
  Masas : S-Function  FunctionName=sinertia  Parameters=dyn  PortCounts=[]  SFunctionModules=''
  Mux : Mux  Inputs=2
      settings: DisplayOption=none
  M (q)·In : Outport  Port=1  InitialOutput=0
  wires:
  Mux/1 -> Masas/1
  q/1 -> Mux/1
  In/1 -> Mux/2
  Masas/1 -> M (q)·In/1

== system HEMERO/Robots manipuladores base fija/Control basado en el modelo/Par Computado/Ejemplos/Ejemplo H.5.3/Estimada3 ==
  q : Inport  Port=1  PortWidth=-1  SampleTime=-1  DataType=auto
      settings: SignalType=auto
  q' : Inport  Port=2  PortWidth=-1  SampleTime=-1  DataType=auto
      settings: SignalType=auto
  Centrífugos y Coriolis : S-Function  FunctionName=scoriolis  Parameters=dyn  PortCounts=[]  SFunctionModules=''
  Mux : Mux  Inputs=2
      settings: DisplayOption=none
  V (q,q') : Outport  Port=1  InitialOutput=0
  wires:
  Mux/1 -> Centrífugos y Coriolis/1
  q/1 -> Mux/1
  q'/1 -> Mux/2
  Centrífugos y Coriolis/1 -> V (q,q')/1

== system HEMERO/Robots manipuladores base fija/Control basado en el modelo/Par Computado/Ejemplos/Ejemplo H.5.3/Real1 ==
  q : Inport  Port=1  PortWidth=-1  SampleTime=-1  DataType=auto
      settings: SignalType=auto
  q' : Inport  Port=2  PortWidth=-1  SampleTime=-1  DataType=auto
      settings: SignalType=auto
  Centrífugos y Coriolis : S-Function  FunctionName=scoriolis  Parameters=dyn  PortCounts=[]  SFunctionModules=''
  Mux : Mux  Inputs=2
      settings: DisplayOption=none
  V (q,q') : Outport  Port=1  InitialOutput=0
  wires:
  Mux/1 -> Centrífugos y Coriolis/1
  q/1 -> Mux/1
  q'/1 -> Mux/2
  Centrífugos y Coriolis/1 -> V (q,q')/1

== system HEMERO/Robots manipuladores base fija/Control basado en el modelo/Par Computado/Ejemplos/Ejemplo H.5.3/Real2 ==
  q : Inport  Port=1  PortWidth=-1  SampleTime=-1  DataType=auto
      settings: SignalType=auto
  Gravedad : S-Function  FunctionName=sgravity  Parameters=dyn,grav  PortCounts=[]  SFunctionModules=''
  G (q) : Outport  Port=1  InitialOutput=0
  wires:
  q/1 -> Gravedad/1
  Gravedad/1 -> G (q)/1

== system HEMERO/Robots manipuladores base fija/Control basado en el modelo/Par Computado/Ejemplos/Ejemplo H.5.3/Real3 ==
  q : Inport  Port=1  PortWidth=-1  SampleTime=-1  DataType=auto
      settings: SignalType=auto
  In : Inport  Port=2  PortWidth=-1  SampleTime=-1  DataType=auto
      settings: SignalType=auto
  Masas : S-Function  FunctionName=sminv  Parameters=dyn  PortCounts=[]  SFunctionModules=''
  Mux : Mux  Inputs=2
      settings: DisplayOption=none
  M(q)^(-1) · In : Outport  Port=1  InitialOutput=0
  wires:
  Mux/1 -> Masas/1
  q/1 -> Mux/1
  In/1 -> Mux/2
  Masas/1 -> M(q)^(-1) · In/1

== system HEMERO/Robots manipuladores base fija/Control basado en el modelo/Par Computado/Ejemplos/Ejemplo H.5.4/Control PID ==
  note: e
  note: e'
  qd : Inport  Port=1  PortWidth=-1  SampleTime=-1  DataType=auto
      settings: SignalType=auto
  q : Inport  Port=2  PortWidth=-1  SampleTime=-1  DataType=auto
      settings: SignalType=auto
  qd' : Inport  Port=3  PortWidth=-1  SampleTime=-1  DataType=auto
      settings: SignalType=auto
  q' : Inport  Port=4  PortWidth=-1  SampleTime=-1  DataType=auto
      settings: SignalType=auto
  qd'' : Inport  Port=5  PortWidth=-1  SampleTime=-1  DataType=auto
      settings: SignalType=auto
  Integrator : Integrator  ExternalReset=none  InitialConditionSource=internal  InitialCondition=0  LimitOutput=off  UpperSaturationLimit=inf  LowerSaturationLimit=-inf  ShowSaturationPort=off  ShowStatePort=off  AbsoluteTolerance=auto
  Ki : HEMERO/Robots manipuladores base fija/Control basado en el modelo/Par Computado/Control PID/Ki  MaskParam1=Ki
  Kp : HEMERO/Robots manipuladores base fija/Control basado en el modelo/Par Computado/Control PID/Kp  MaskParam1=Kp
  Kv : HEMERO/Robots manipuladores base fija/Control basado en el modelo/Par Computado/Control PID/Kv  MaskParam1=Kv
  Sum : Sum  Inputs=+-  SaturateOnIntegerOverflow=on
  Sum1 : Sum  Inputs=+-  SaturateOnIntegerOverflow=on
  Sum2 : Sum  Inputs=++++  SaturateOnIntegerOverflow=on
  tau_r : Outport  Port=1  InitialOutput=0
  wires:
  Sum2/1 -> tau_r/1
  Sum1/1 -> Kv/1
  q'/1 -> Sum1/2
  qd'/1 -> Sum1/1
  q/1 -> Sum/2
  qd/1 -> Sum/1
  qd''/1 -> Sum2/4
  Kv/1 -> Sum2/3
  Kp/1 -> Sum2/2
  Sum/1 -> Kp/1, Ki/1
  Ki/1 -> Integrator/1
  Integrator/1 -> Sum2/1

== system HEMERO/Robots manipuladores base fija/Control basado en el modelo/Par Computado/Ejemplos/Ejemplo H.5.4/Estimada1 ==
  q : Inport  Port=1  PortWidth=-1  SampleTime=-1  DataType=auto
      settings: SignalType=auto
  Gravedad : S-Function  FunctionName=sgravity  Parameters=dyn,grav  PortCounts=[]  SFunctionModules=''
  G (q) : Outport  Port=1  InitialOutput=0
  wires:
  q/1 -> Gravedad/1
  Gravedad/1 -> G (q)/1

== system HEMERO/Robots manipuladores base fija/Control basado en el modelo/Par Computado/Ejemplos/Ejemplo H.5.4/Estimada2 ==
  q : Inport  Port=1  PortWidth=-1  SampleTime=-1  DataType=auto
      settings: SignalType=auto
  In : Inport  Port=2  PortWidth=-1  SampleTime=-1  DataType=auto
      settings: SignalType=auto
  Masas : S-Function  FunctionName=sinertia  Parameters=dyn  PortCounts=[]  SFunctionModules=''
  Mux : Mux  Inputs=2
      settings: DisplayOption=none
  M (q)·In : Outport  Port=1  InitialOutput=0
  wires:
  Mux/1 -> Masas/1
  q/1 -> Mux/1
  In/1 -> Mux/2
  Masas/1 -> M (q)·In/1

== system HEMERO/Robots manipuladores base fija/Control basado en el modelo/Par Computado/Ejemplos/Ejemplo H.5.4/Estimada3 ==
  q : Inport  Port=1  PortWidth=-1  SampleTime=-1  DataType=auto
      settings: SignalType=auto
  q' : Inport  Port=2  PortWidth=-1  SampleTime=-1  DataType=auto
      settings: SignalType=auto
  Centrífugos y Coriolis : S-Function  FunctionName=scoriolis  Parameters=dyn  PortCounts=[]  SFunctionModules=''
  Mux : Mux  Inputs=2
      settings: DisplayOption=none
  V (q,q') : Outport  Port=1  InitialOutput=0
  wires:
  Mux/1 -> Centrífugos y Coriolis/1
  q/1 -> Mux/1
  q'/1 -> Mux/2
  Centrífugos y Coriolis/1 -> V (q,q')/1

== system HEMERO/Robots manipuladores base fija/Control basado en el modelo/Par Computado/Ejemplos/Ejemplo H.5.4/Real1 ==
  q : Inport  Port=1  PortWidth=-1  SampleTime=-1  DataType=auto
      settings: SignalType=auto
  q' : Inport  Port=2  PortWidth=-1  SampleTime=-1  DataType=auto
      settings: SignalType=auto
  Centrífugos y Coriolis : S-Function  FunctionName=scoriolis  Parameters=dyn  PortCounts=[]  SFunctionModules=''
  Mux : Mux  Inputs=2
      settings: DisplayOption=none
  V (q,q') : Outport  Port=1  InitialOutput=0
  wires:
  Mux/1 -> Centrífugos y Coriolis/1
  q/1 -> Mux/1
  q'/1 -> Mux/2
  Centrífugos y Coriolis/1 -> V (q,q')/1

== system HEMERO/Robots manipuladores base fija/Control basado en el modelo/Par Computado/Ejemplos/Ejemplo H.5.4/Real2 ==
  q : Inport  Port=1  PortWidth=-1  SampleTime=-1  DataType=auto
      settings: SignalType=auto
  Gravedad : S-Function  FunctionName=sgravity  Parameters=dyn,grav  PortCounts=[]  SFunctionModules=''
  G (q) : Outport  Port=1  InitialOutput=0
  wires:
  q/1 -> Gravedad/1
  Gravedad/1 -> G (q)/1

== system HEMERO/Robots manipuladores base fija/Control basado en el modelo/Par Computado/Ejemplos/Ejemplo H.5.4/Real3 ==
  q : Inport  Port=1  PortWidth=-1  SampleTime=-1  DataType=auto
      settings: SignalType=auto
  In : Inport  Port=2  PortWidth=-1  SampleTime=-1  DataType=auto
      settings: SignalType=auto
  Masas : S-Function  FunctionName=sminv  Parameters=dyn  PortCounts=[]  SFunctionModules=''
  Mux : Mux  Inputs=2
      settings: DisplayOption=none
  M(q)^(-1) · In : Outport  Port=1  InitialOutput=0
  wires:
  Mux/1 -> Masas/1
  q/1 -> Mux/1
  In/1 -> Mux/2
  Masas/1 -> M(q)^(-1) · In/1

== system HEMERO/Robots manipuladores base fija/Modelo Dinámico/Ejemplos/Ejemplo H.4.2/Trayectorias articulares/Inversa de la matriz de masas ==
  q : Inport  Port=1  PortWidth=-1  SampleTime=-1  DataType=auto
      settings: SignalType=auto
  In : Inport  Port=2  PortWidth=-1  SampleTime=-1  DataType=auto
      settings: SignalType=auto
  Masas : S-Function  FunctionName=sminv  Parameters=dyn  PortCounts=[]  SFunctionModules=''
  Mux : Mux  Inputs=2
      settings: DisplayOption=none
  M(q)^(-1) · In : Outport  Port=1  InitialOutput=0
  wires:
  Masas/1 -> M(q)^(-1) · In/1
  In/1 -> Mux/2
  q/1 -> Mux/1
  Mux/1 -> Masas/1

== system HEMERO/Robots manipuladores base fija/Modelo Dinámico/Ejemplos/Ejemplo H.4.2/Trayectorias articulares/Modelo de fricciones ==
  q' : Inport  Port=1  PortWidth=-1  SampleTime=-1  DataType=auto
      settings: SignalType=auto
  Fricciones : S-Function  FunctionName=sfriction  Parameters=G,b,tcp,tcm  PortCounts=[]  SFunctionModules=''
  tau_f : Outport  Port=1  InitialOutput=0
  wires:
  Fricciones/1 -> tau_f/1
  q'/1 -> Fricciones/1

== system HEMERO/Robots manipuladores base fija/Modelo Dinámico/Ejemplos/Ejemplo H.4.2/Trayectorias articulares/Términos gravitatorios ==
  q : Inport  Port=1  PortWidth=-1  SampleTime=-1  DataType=auto
      settings: SignalType=auto
  Gravedad : S-Function  FunctionName=sgravity  Parameters=dyn,grav  PortCounts=[]  SFunctionModules=''
  G (q) : Outport  Port=1  InitialOutput=0
  wires:
  Gravedad/1 -> G (q)/1
  q/1 -> Gravedad/1

== system HEMERO/Robots manipuladores base fija/Modelo Dinámico/Ejemplos/Ejemplo H.4.2/Trayectorias articulares/Términos centrífugos y de Coriolis ==
  q : Inport  Port=1  PortWidth=-1  SampleTime=-1  DataType=auto
      settings: SignalType=auto
  q' : Inport  Port=2  PortWidth=-1  SampleTime=-1  DataType=auto
      settings: SignalType=auto
  Centrífugos y Coriolis : S-Function  FunctionName=scoriolis  Parameters=dyn  PortCounts=[]  SFunctionModules=''
  Mux : Mux  Inputs=2
      settings: DisplayOption=none
  V (q,q') : Outport  Port=1  InitialOutput=0
  wires:
  Centrífugos y Coriolis/1 -> V (q,q')/1
  q'/1 -> Mux/2
  q/1 -> Mux/1
  Mux/1 -> Centrífugos y Coriolis/1

== system HEMERO/Robots móviles/Control de robots móviles/Métodos basados en Teoría de Control/Seguimiento de caminos/Ejemplos/Ejemplo H.6.4 ==
  Constant1 : Constant  Value=1
  Seguimiento de caminos (control lineal) : Subsystem  mask(Seguimiento de caminos empleando una ley de control lineal){x_inicial=0, y_inicial=0, phi_inicial=0, K1=K1, K2=K2, x_camino=x_camino, y_camino=y_camino}
      mask prompts: x_inicial "Coordenada x inicial del móvil:"; y_inicial "Coordenada y inicial del móvil:"; phi_inicial "Valor inicial de la orientación del móvil:"; K1 "Parámetro K1:"; K2 "Parámetro K2:"; x_camino "Vector con las coordenadas x del camino:"; y_camino "Vector con las coordenadas y del camino:"
      mask help:
      | Este bloque permite simular una estrategia de control lineal para el seguimiento de caminos.
      | A la entrada se dispone de la velocidad del vehículo en cada instante y mediante los parámetros es posible introducir las coordenadas (x,y) del camino. A la salida se obtienen las coordenadas y orientación del vehículo en cada instante.
      mask init:
      | der_x = diff(x_camino);
      | der_y = diff(y_camino);
  To Workspace3 : ToWorkspace  VariableName=x_v  SampleTime=-1  SaveFormat=Matrix
  To Workspace4 : ToWorkspace  VariableName=y_v  SampleTime=-1  SaveFormat=Matrix
  To Workspace5 : ToWorkspace  VariableName=phi_v  SampleTime=-1  SaveFormat=Matrix
  wires:
  Constant1/1 -> Seguimiento de caminos (control lineal)/1(v)
  Seguimiento de caminos (control lineal)/1(x_vehículo) -> To Workspace3/1
  Seguimiento de caminos (control lineal)/3(phi_vehículo) -> To Workspace5/1
  Seguimiento de caminos (control lineal)/2(y_vehículo) -> To Workspace4/1

== system HEMERO/Robots móviles/Control de robots móviles/Métodos basados en Teoría de Control/Seguimiento de caminos/Ejemplos/Ejemplo H.6.5 ==
  Constant1 : Constant  Value=1
  Seguimiento de caminos (control no lineal) : Subsystem  mask(Seguimiento de caminos empleando una ley de control no lineal){x_inicial=0, y_inicial=0, phi_inicial=0, K1=K1, K2=K2, x_camino=x_camino, y_camino=y_camino}
      mask prompts: x_inicial "Coordenada x inicial del móvil:"; y_inicial "Coordenada y inicial del móvil:"; phi_inicial "Valor inicial de la orientación del móvil:"; K1 "Parámetro K1:"; K2 "Parámetro K2:"; x_camino "Vector con las coordenadas x del camino:"; y_camino "Vector con las coordenadas y del camino:"
      mask help:
      | Este bloque permite simular una estrategia de control no lineal para el seguimiento de caminos.
      | A la entrada se dispone de la velocidad del vehículo en cada instante y mediante los parámetros es posible introducir las coordenadas (x,y) del camino. A la salida se obtienen las coordenadas y orientación del vehículo en cada instante.
      mask init:
      | der_x = diff(x_camino);
      | der_y = diff(y_camino);
  To Workspace3 : ToWorkspace  VariableName=x_v  SampleTime=-1  SaveFormat=Matrix
  To Workspace4 : ToWorkspace  VariableName=y_v  SampleTime=-1  SaveFormat=Matrix
  To Workspace5 : ToWorkspace  VariableName=phi_v  SampleTime=-1  SaveFormat=Matrix
  wires:
  Constant1/1 -> Seguimiento de caminos (control no lineal)/1(v)
  Seguimiento de caminos (control no lineal)/1(x_vehículo) -> To Workspace3/1
  Seguimiento de caminos (control no lineal)/3(phi_vehículo) -> To Workspace5/1
  Seguimiento de caminos (control no lineal)/2(y_vehículo) -> To Workspace4/1

== system HEMERO/Robots móviles/Control de robots móviles/Métodos basados en Teoría de Control/Seguimiento de caminos/Seguimiento de caminos (control lineal)/Configuracion síncrona ==
  v : Inport  Port=1  PortWidth=-1  SampleTime=-1  DataType=auto
      settings: SignalType=auto
  w : Inport  Port=2  PortWidth=-1  SampleTime=-1  DataType=auto
      settings: SignalType=auto
  Fcn : Fcn  Expr=-sin(u)
  Fcn1 : Fcn  Expr=cos(u)
  Integrator : Integrator  ExternalReset=none  InitialConditionSource=internal  InitialCondition=phi_inicial  LimitOutput=off  UpperSaturationLimit=inf  LowerSaturationLimit=-inf  ShowSaturationPort=off  ShowStatePort=off  AbsoluteTolerance=auto
  Integrator1 : Integrator  ExternalReset=none  InitialConditionSource=internal  InitialCondition=x_inicial  LimitOutput=off  UpperSaturationLimit=inf  LowerSaturationLimit=-inf  ShowSaturationPort=off  ShowStatePort=off  AbsoluteTolerance=auto
  Integrator2 : Integrator  ExternalReset=none  InitialConditionSource=internal  InitialCondition=y_inicial  LimitOutput=off  UpperSaturationLimit=inf  LowerSaturationLimit=-inf  ShowSaturationPort=off  ShowStatePort=off  AbsoluteTolerance=auto
  Product : Product  Inputs=2  SaturateOnIntegerOverflow=on
  Product1 : Product  Inputs=2  SaturateOnIntegerOverflow=on
  x_vehículo : Outport  Port=1
  y_vehículo : Outport  Port=2
  phi_vehículo : Outport  Port=3
  wires:
  Product1/1 -> Integrator2/1
  Product/1 -> Integrator1/1
  Fcn/1 -> Product/2
  Integrator/1 -> Fcn/1, Fcn1/1, phi_vehículo/1
  Integrator1/1 -> x_vehículo/1
  Integrator2/1 -> y_vehículo/1
  v/1 -> Product/1, Product1/1
  w/1 -> Integrator/1
  Fcn1/1 -> Product1/2

== system HEMERO/Robots móviles/Control de robots móviles/Métodos basados en Teoría de Control/Seguimiento de caminos/Seguimiento de caminos (control lineal)/Controlador lineal ==
  fi_gorro : Inport  Port=1  PortWidth=-1  SampleTime=-1  DataType=auto
      settings: SignalType=auto
  v : Inport  Port=2  PortWidth=-1  SampleTime=-1  DataType=auto
      settings: SignalType=auto
  epsilon : Inport  Port=3  PortWidth=-1  SampleTime=-1  DataType=auto
      settings: SignalType=auto
  Abs : Abs
  Gain : Gain  Gain=K1  SaturateOnIntegerOverflow=on
  Gain1 : Gain  Gain=K2  SaturateOnIntegerOverflow=on
  Product : Product  Inputs=2  SaturateOnIntegerOverflow=on
  Product1 : Product  Inputs=2  SaturateOnIntegerOverflow=on
  Sum : Sum  Inputs=--  SaturateOnIntegerOverflow=on
  u_cont : Outport  Port=1  InitialOutput=0
  wires:
  fi_gorro/1 -> Gain1/1
  Sum/1 -> u_cont/1
  epsilon/1 -> Gain/1
  Product1/1 -> Sum/2
  Product/1 -> Sum/1
  Abs/1 -> Product1/2
  Gain1/1 -> Product1/1
  v/1 -> Abs/1, Product/2
  Gain/1 -> Product/1
